simulink model "linmodel_eq1_discr2"  (R2019a)
settings: Solver=VariableStepAuto  StartTime=0.0  StopTime=30  RelTol=1e-3
InitFcn:
  | lin_discr_model
undefined symbols (not defined in the file): A_eq1_d, B_eq1_d, C_eq1_d, D_eq1_d, DiscIntNeverNeededParam, Discrete, Time, Ts
libraries: ctrlSharedLib x1
settings Model: Creator=jessi  LastModifiedBy=jessi

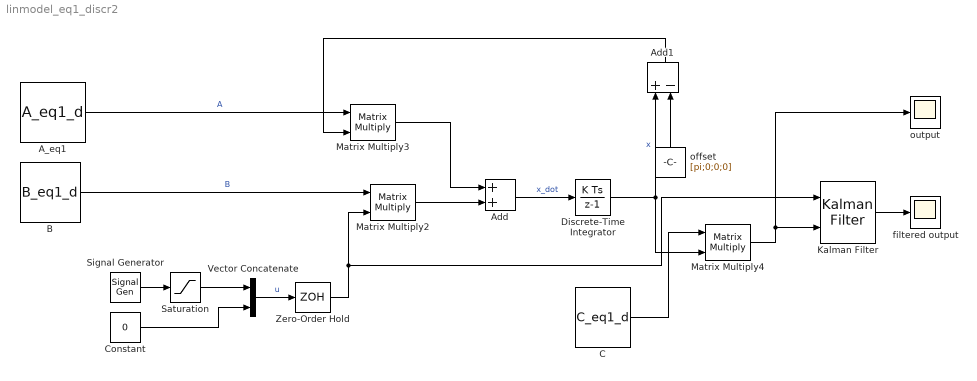
== system linmodel_eq1_discr2 ==
  A_eq1 : Constant  Value=A_eq1_d
  Add : Sum
  Add1 : Sum  Inputs=+-
  B : Constant  Value=B_eq1_d
  C : Constant  Value=C_eq1_d
  Constant : Constant  Value=0
  Discrete-Time Integrator : DiscreteIntegrator  InitialCondition=[pi;0;0;0]  SampleTime=Ts  ICPrevOutput=DiscIntNeverNeededParam  ICPrevScaledInput=DiscIntNeverNeededParam
  Kalman Filter : ctrlSharedLib/Kalman Filter  TimeDomain=Discrete-Time  UseCurrentEstimator=on  ModelSource=Individual A, B, C, D matrices  ModelSourceVariable=ss(0.95,1,1,0,1)  A=A_eq1_d  B=B_eq1_d  C=C_eq1_d  D=D_eq1_d  NumberOfStates=1  NumberOfInputs=1  NumberOfOutputs=1  InitialEstimateSource=Dialog  X0=[pi;0;0;0]  P0=10  UseK=off  UseGH=off  NumberOfProcessNoiseInputs=1  G=1  TimeInvariantG=on  H=0  TimeInvariantH=on  Q=diag([1, 1, 10, 10])  TimeInvariantQ=on  R=diag([0.1, 0.1])  TimeInvariantR=on  N=0  TimeInvariantN=on  AddInputPort=on  AddEnablePort=off  OutputEstimatedY=off  OutputP=off  Ts=Ts
      settings: SourceProductBaseCode=CT
  Matrix Multiply2 : Product  Multiplication=Matrix(*)
  Matrix Multiply3 : Product  Multiplication=Matrix(*)
  Matrix Multiply4 : Product  Multiplication=Matrix(*)
  Saturation : Saturate  UpperLimit=1  LowerLimit=-1
  Signal Generator : SignalGenerator  WaveForm=square  Amplitude=0.3
  Vector Concatenate : Concatenate
  Zero-Order Hold : ZeroOrderHold  SampleTime=Ts
  filtered output : Scope
  offset : Constant  Value=[pi;0;0;0]  SampleTime=-1
  output : Scope
  wires:
  B/1 -> Matrix Multiply2/1  "B"
  Matrix Multiply2/1 -> Add/2
  A_eq1/1 -> Matrix Multiply3/1  "A"
  Add/1 -> Discrete-Time Integrator/1  "x_dot"
  Discrete-Time Integrator/1 -> Matrix Multiply4/2, Add1/1  "x"
  Matrix Multiply3/1 -> Add/1
  Matrix Multiply4/1 -> Kalman Filter/2, output/1
  Signal Generator/1 -> Saturation/1
  Constant/1 -> Vector Concatenate/2
  Vector Concatenate/1 -> Zero-Order Hold/1  "u"
  C/1 -> Matrix Multiply4/1
  Saturation/1 -> Vector Concatenate/1
  Kalman Filter/1 -> filtered output/1
  offset/1 -> Add1/2
  Add1/1 -> Matrix Multiply3/2
  Zero-Order Hold/1 -> Kalman Filter/1, Matrix Multiply2/2
